simulink model "p14"  (R2023a)
settings: Solver=VariableStepAuto  StartTime=0.0  StopTime=10.0  RelTol=1e-3
libraries: dspsnks4 x1, dspfdesign x1, simulink x1
settings Model: Creator=mcconncm  LastModifiedBy=mcconncm

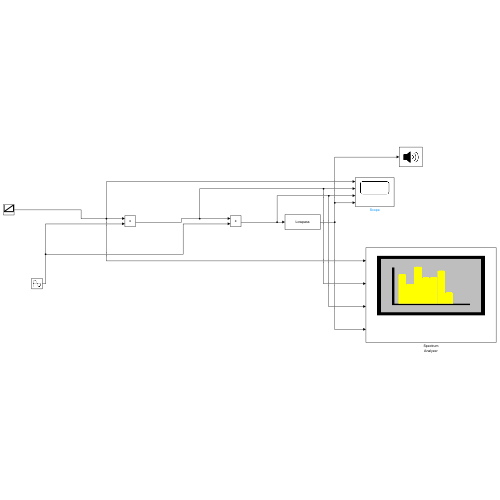
[thumbnail: Simulink's stored preview of the top-level diagram]
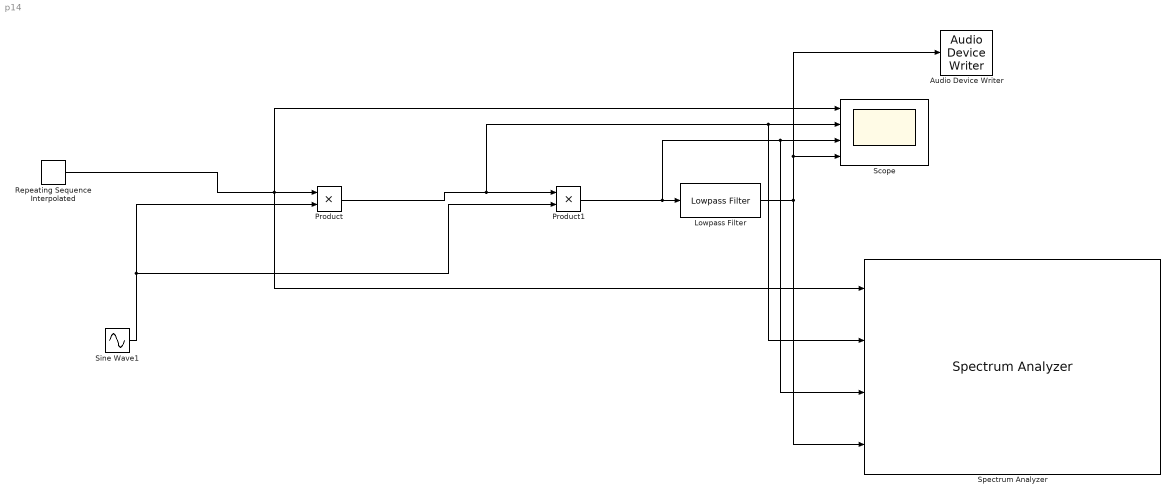
== system p14 ==
  Audio Device Writer : dspsnks4/Audio Device Writer  Driver=DirectSound  Device=Default  InheritSampleRate=on  SampleRate=44100  BitDepth=16-bit integer  BufferSize=4096  NumBuffers=10  DefaultOutputChannelMapping=on  OutputChannelMapping=1:2  OutputNumUnderrunSamples=off  DriverIdx=1  DeviceWarnFlag=''
  Lowpass Filter : dspfdesign/Lowpass Filter  FilterType=FIR  DesignForMinimumOrder=on  FilterOrder=50  PassbandFrequency=2000  StopbandFrequency=3000  PassbandRipple=1  StopbandAttenuation=60  SampleRate=44100  SimulateUsing=Interpreted execution  roundingMode=Floor  coeffsDataTypeStr=fixdt(1,16)
  Product : Product
  Product1 : Product
  Repeating Sequence Interpolated : simulink/Sources/Repeating Sequence Interpolated  OutValues=[0 1 0]  TimeValues=[0 .01 .01001]  LookUpMeth=Interpolation-Use End Values  tsamp=1/44100  OutMin=[]  OutMax=[]  OutDataTypeStr=double  OutputDataTypeScalingMode=double  OutDataType=fixdt(0,8)  OutScaling=2^-10
  Scope : Scope  NumInputPorts=4
  Sine Wave1 : Sin  Frequency=10000*2*pi  SampleTime=1/44100
  Spectrum Analyzer : SpectrumAnalyzer  NumInputPorts=4  WindowPosition=[560.000000,290.000000,800.000000,500.000000,]  Visible=on  ScopeFrameLocation=window  Span=44100  StartFrequency=-22050  StopFrequency=22050  YLimits=[-206.00026027,49.53269429]  ColorLimits=[-20 80]  ShowLegend=on  DefaultConfigurationName=spbscopes.SpectrumAnalyzerBlockCfg  IsFrequencyInputMode=0  FrequencyVectorPort=0  FrequencyVectorFromPort=0  FrequencyInputRBWPort=0  FrequencyInputRBWFromPort=0
  wires:
  Sine Wave1/1 -> Product1/2, Product/2
  Repeating Sequence Interpolated/1 -> Scope/1, Spectrum Analyzer/1, Product/1
  Product1/1 -> Scope/3, Spectrum Analyzer/3, Lowpass Filter/1
  Product/1 -> Scope/2, Spectrum Analyzer/2, Product1/1
  Lowpass Filter/1 -> Scope/4, Audio Device Writer/1, Spectrum Analyzer/4
